simulink model "openLoop_compat"  (Simulink 8.7)
settings: Solver=ode45  StartTime=0.0  StopTime=t_max  RelTol=1e-3
libraries: simulink x1, cjt_library_models x1
settings Model: Creator=joern  LastModifiedBy=J�rn
settings DebuggingCC: UnderspecifiedInitializationDetection=Simplified  MergeDetectMultiDrivingBlocksExec=error  SolverPrmCheckMsg=warning
settings ConfigComp: CovModelRefEnable=off  CovSFcnEnable=off

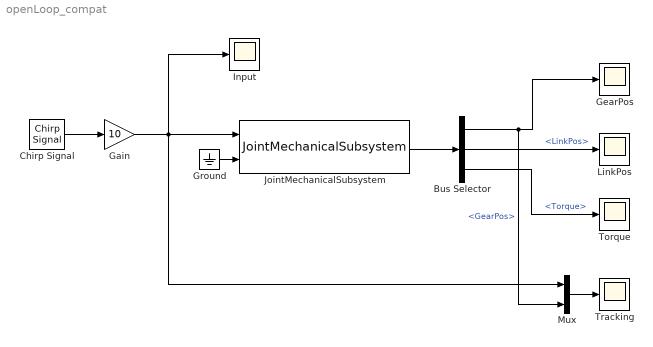
== system openLoop_compat ==
  Bus Selector : BusSelector  OutputSignals=GearPos,LinkPos,Torque
  Chirp Signal : simulink/Sources/Chirp Signal  f1=0.1  T=60  f2=60
  Gain : Gain  Gain=10
  GearPos : Scope
  Ground : Ground
  Input : Scope
  JointMechanicalSubsystem : cjt_library_models/Joint models/JointMechanicalSubsystem  jointObj=jointObj  fc_vel=499  fc_torque=499  input_delay=1  output_delay=1  quantize=on  quantize_bits=19  input_noise_enabled=off  output_noise_enabled=off  var_u=0.12^2  var_y=1.8e-10
  LinkPos : Scope
  Mux : Mux  Inputs=2
  Torque : Scope
  Tracking : Scope
  wires:
  JointMechanicalSubsystem/1 -> Bus Selector/1
  Bus Selector/2 -> LinkPos/1  "<LinkPos>"
  Bus Selector/3 -> Torque/1  "<Torque>"
  Mux/1 -> Tracking/1
  Bus Selector/1 -> Mux/2, GearPos/1  "<GearPos>"
  Chirp Signal/1 -> Gain/1
  Gain/1 -> JointMechanicalSubsystem/1, Input/1, Mux/1
  Ground/1 -> JointMechanicalSubsystem/2
